simulink model "beachball_ver2"  (R2022b)
settings: Solver=VariableStepAuto  StartTime=0.0  StopTime=20  RelTol=1e-3
libraries: VACLib x6
settings Model: Creator=KarlO  LastModifiedBy=KarlO

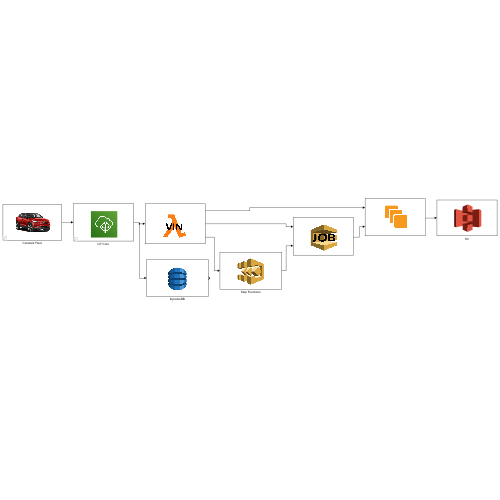
[thumbnail: Simulink's stored preview of the top-level diagram]
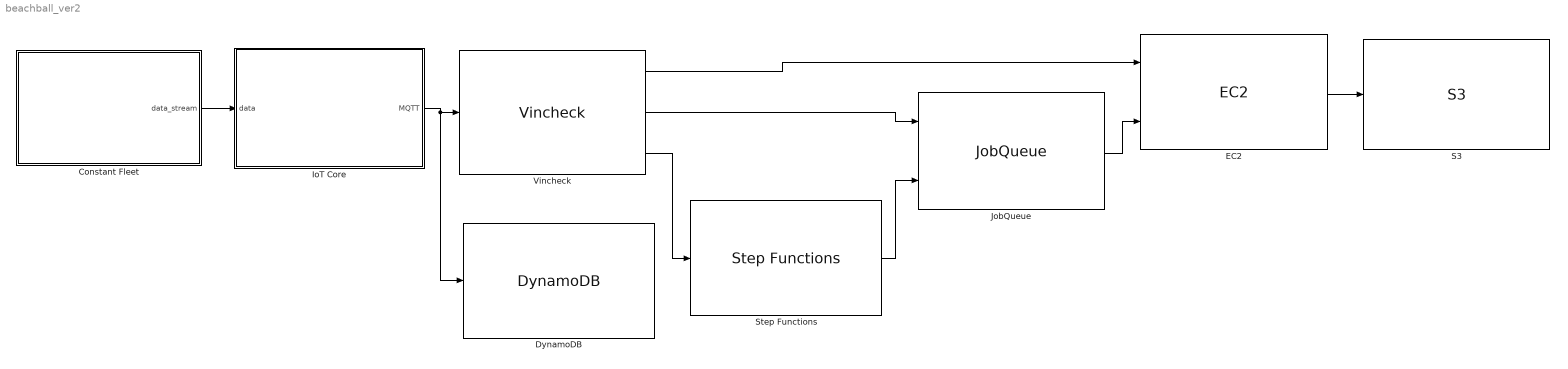
== system beachball_ver2 ==
  Constant Fleet : Subsystem  AncestorBlock=VACLib/Vehicle Components/Constant Fleet
      settings: LibrarySourceBlock=VACLib/Vehicle Components/Constant Fleet
      mask Display: image('C:\Users\KarlO\architectural-tradeoff-analysis\DCA-simulator\Volvo Architecture\VAC library\Images\VAC\cc9459c7a9e4acd4eb37509497aa20bf.png',[40,10,125,100]); % Use "Edit Image" on toolstrip to change.
  DynamoDB : VACLib/AWS Components/DynamoDB  SystemSampleTime=-1  VariantActivationTime=update diagram  Latency=0  AutoFrameSizeCalculation=off
      settings: SourceProductName=Volvo Architechture Components
  EC2 : VACLib/AWS Components/EC2  SystemSampleTime=-1  VariantActivationTime=update diagram  Latency=0  AutoFrameSizeCalculation=off
      settings: SourceProductName=Volvo Architechture Components
  IoT Core : Subsystem  AncestorBlock=VACLib/AWS Components/IoT Core
      settings: LibrarySourceBlock=VACLib/AWS Components/IoT Core
      mask Display: image('C:\Users\KarlO\architectural-tradeoff-analysis\DCA-simulator\Volvo Architecture\VAC library\Images\VAC\AWS-IoT-Core.png',[60,12,90,90]); % Use "Edit Image" on toolstrip to change.
  JobQueue : VACLib/AWS Components/JobQueue  SystemSampleTime=-1  VariantActivationTime=update diagram  Latency=0  AutoFrameSizeCalculation=off
      settings: SourceProductName=Volvo Architechture Components
  S3 : VACLib/AWS Components/S3  SystemSampleTime=-1  VariantActivationTime=update diagram  Latency=0  AutoFrameSizeCalculation=off
      settings: SourceProductName=Volvo Architechture Components
  Step Functions : VACLib/AWS Components/Step Functions  SystemSampleTime=-1  VariantActivationTime=update diagram  Latency=0  AutoFrameSizeCalculation=off
      settings: SourceProductName=Volvo Architechture Components
  Vincheck : VACLib/AWS Components/Vincheck  SystemSampleTime=-1  VariantActivationTime=update diagram  Latency=0  AutoFrameSizeCalculation=off
      settings: SourceProductName=Volvo Architechture Components
  wires:
  Constant Fleet/1(data_stream) -> IoT Core/1(data)
  IoT Core/1(MQTT) -> DynamoDB/1, Vincheck/1
  Step Functions/1 -> JobQueue/2
  Vincheck/1 -> EC2/1
  EC2/1 -> S3/1
  Vincheck/2 -> JobQueue/1
  Vincheck/3 -> Step Functions/1
  JobQueue/1 -> EC2/2

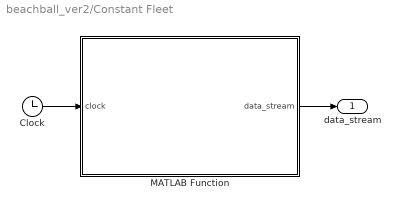
== system beachball_ver2/Constant Fleet ==
  Clock : Clock
  MATLAB Function : MATLAB Function  TreatAsAtomicUnit=on
  data_stream : Outport
  wires:
  Clock/1 -> MATLAB Function/1(clock)
  MATLAB Function/1(data_stream) -> data_stream/1

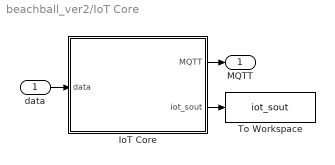
== system beachball_ver2/IoT Core ==
  data : Inport
  IoT Core : MATLAB Function  TreatAsAtomicUnit=on
  To Workspace : ToWorkspace  VariableName=iot_sout  SaveFormat=Timeseries  SampleTime=-1
  MQTT : Outport
  wires:
  IoT Core/2(iot_sout) -> To Workspace/1
  data/1 -> IoT Core/1(data)
  IoT Core/1(MQTT) -> MQTT/1

== matlab function beachball_ver2/Constant Fleet/MATLAB Function ==
  data: clock input; data_stream output
function data_stream  = fcn(clock)

persistent out;
persistent last_tick;
persistent data_to_send;

message_size = 1;
car_cache = 1;
fleet_size = 1000;
simulation_time = 10;

if isempty(out)
    out = 0;
    data_to_send = (message_size*fleet_size*simulation_time);
    last_tick = 0;
end

tick = clock;
passed_time = tick-last_tick;
last_tick = tick;

send_this_tick = (data_to_send/simulation_time)*passed_time;

to_send = floor(send_this_tick/(car_cache*message_size));

if tick >= simulation_time
    out = data_to_send;
else
    out = out + (to_send*car_cache*message_size);
end

data_stream = [out,(car_cache*message_size), fleet_size, simulation_time];

== matlab function beachball_ver2/IoT Core/IoT Core ==
  data: data input; MQTT output; iot_sout output
function [MQTT,iot_sout]= iot_core(data)

data_received = data(1);
data_package_size = data(2);
no_of_devices = data(3);
simulation_time = data(4);

no_of_messages_received =  round(data_received/data_package_size);
billable_messages = ceil(data_package_size/(5/1000));
messages_sent = no_of_messages_received * billable_messages;

connectivity_charges = (simulation_time/60) * no_of_devices * (0.08/1000000);

messaging_charges = messages_sent *  0.000001;
cost = messaging_charges + connectivity_charges;

iot_sout = [0,cost,0,0];

MQTT = data;
